simulink model "test"  (R2025b)
settings: Solver=ode5  StartTime=0.0  StopTime=40  RelTol=1e-3
StartFcn:
  | MaxMissedTicks = 99^100;
  | SampleTime = 0.01;
undefined symbols (not defined in the file or in its folder): National_Instruments, PCI
libraries: sldrtlib x6, simulink x1
settings Model: Creator=labadmin  LastModifiedBy=aie4-26
settings HardwareCC: ProdBitPerLong=64.0  ProdHWDeviceType=Intel->x86-64 (Linux 64)
settings RTWCC: SystemTargetFile=sldrt.tlc  TemplateMakefile=sldrt.tmf  RTWCompilerOptimization=on  GPUComputeCapability=3.5  Description=Simulink Desktop Real-Time
settings CodeAppCC: MaxIdLength=95.0
settings SimulinkDesktopRealTimeCC: ExtModeTransport=0.0  ExtModeStaticAllocSize=1000000.0  TargetLibSuffix=_sldrt.a  TargetPreCompLibLocation=C:\Program Files\MATLAB\R2025b\toolbox\sldrt\lib\win64  MultiwordLength=2048.0  DynamicStringBufferSize=256.0  ParMdlRefBuildCompliant=on  PreserveMATLABNamespacesInGeneratedCode=on  SubcomponentCodeInterfacePackaging=Reusable function

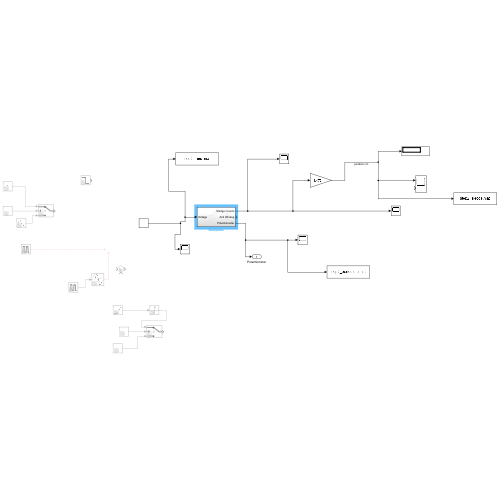
[thumbnail: Simulink's stored preview of the top-level diagram]
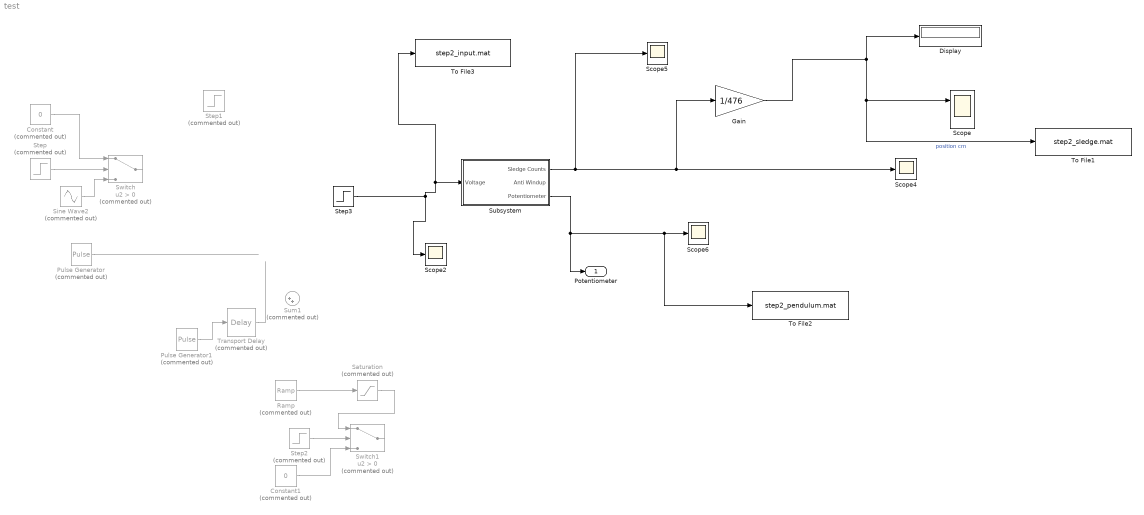
== system test ==
  Constant : Constant  Commented=on  Value=0
  Constant1 : Constant  Commented=on  Value=0
  Display : Display
  Gain : Gain  Gain=1/476
  Pulse Generator : DiscretePulseGenerator  Commented=on  PulseType=Time based  Amplitude=2  Period=10  PulseWidth=3
  Pulse Generator1 : DiscretePulseGenerator  Commented=on  PulseType=Time based  Amplitude=-2  Period=10  PulseWidth=3
  Ramp : simulink/Sources/Ramp  Commented=on  slope=-0.15  start=0  InitialOutput=0
  Saturation : Saturate  Commented=on  UpperLimit=2.2  LowerLimit=-2.2
  Scope : Scope  NumInputPorts=2
      settings: ActiveDisplayYMinimum=-17.820378151260503  ActiveDisplayYMaximum=12.400210084033613  DataLoggingVariableName=ScopeData4
  Scope{2,4..6} (4 alike) : Scope
      Scope2 settings: ActiveDisplayYMinimum=-3.223794053653696  ActiveDisplayYMaximum=6.037574387127588  DataLoggingVariableName=ScopeData6
      Scope4 settings: ActiveDisplayYMinimum=-385.49999999999989  ActiveDisplayYMaximum=3469.5  DataLoggingVariableName=ScopeData8
      Scope5 settings: ActiveDisplayYMinimum=-30594.375  ActiveDisplayYMaximum=3399.3749999999991  DataLoggingVariableName=ScopeData9
      Scope6 settings: ActiveDisplayYMinimum=1.2257068801624322  ActiveDisplayYMaximum=2.6464125172297863  DataLoggingVariableName=ScopeData10
  Sine Wave2 : Sin  Commented=on  Amplitude=1.8  Frequency=4  SampleTime=0
  Step : Step  Commented=on  Time=20  SampleTime=0
  Step1 : Step  Commented=on  Time=0.5  Before=2  After=0  SampleTime=0
  Step2 : Step  Commented=on  Time=10  Before=1  After=0  SampleTime=0
  Step3 : Step  Time=2.0  Before=1.5  After=0  SampleTime=0
  Subsystem : Subsystem
  Sum1 : Sum  Commented=on  Inputs=|++
  Switch : Switch  Commented=on  Criteria=u2 > Threshold  SaturateOnIntegerOverflow=off  InputSameDT=off
  Switch1 : Switch  Commented=on  Criteria=u2 > Threshold  SaturateOnIntegerOverflow=off  InputSameDT=off
  To File1 : ToFile  Filename=step2_sledge.mat  SaveFormat=Timeseries
  To File2 : ToFile  Filename=step2_pendulum.mat  SaveFormat=Timeseries
  To File3 : ToFile  Filename=step2_input.mat  SaveFormat=Timeseries
  Transport Delay : TransportDelay  Commented=on  DelayTime=5
  Potentiometer : Outport
  wires:
  Subsystem/1(Sledge Counts) -> Gain/1, Scope4/1, Scope5/1
  Gain/1 -> Scope/1, To File1/1, Display/1  "position cm"
  Subsystem/3(Potentiometer) -> To File2/1, Scope6/1, Potentiometer/1
  Pulse Generator1/1 -> Transport Delay/1
  Pulse Generator/1 -> ?
  Transport Delay/1 -> ?
  Step/1 -> Switch/2
  Sine Wave2/1 -> Switch/3
  Constant/1 -> Switch/1
  Step3/1 -> To File3/1, Subsystem/1(Voltage), Scope2/1
  Saturation/1 -> Switch1/1
  Step2/1 -> Switch1/2
  Ramp/1 -> Saturation/1
  Constant1/1 -> Switch1/3

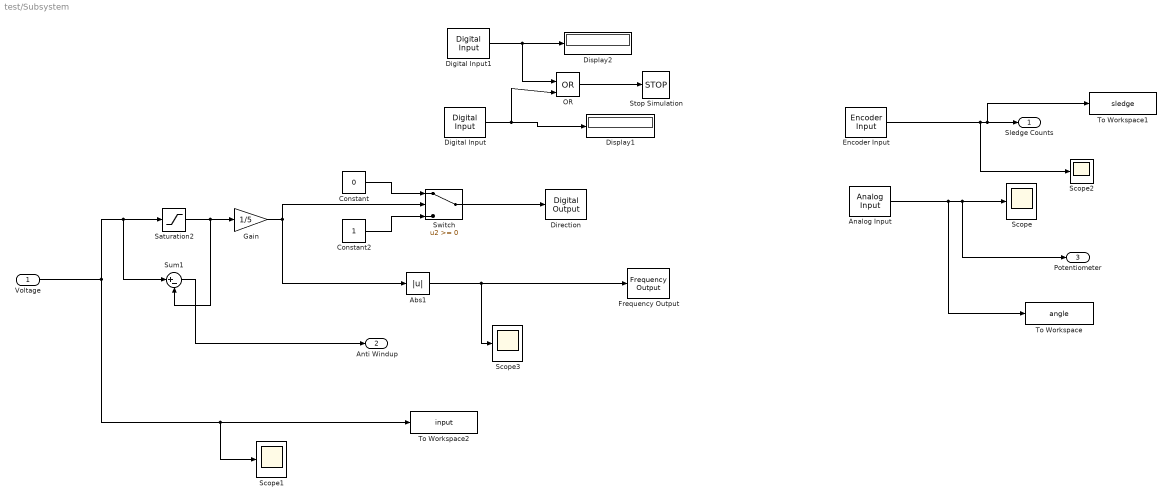
== system test/Subsystem ==
  Voltage : Inport
  Abs1 : Abs  SaturateOnIntegerOverflow=off
  Analog Input : sldrtlib/Analog Input  SampleTime=0.001  MaxMissedTicks=MaxMissedTicks  ShowMissedTicks=off  YieldWhenWaiting=off  DrvName=National_Instruments/PCI-6229  DrvAddress=4294967295  DrvOptions=[1 1 8192 2 3]  Channels=1  RangeMode=1  VoltRange=2  DataType=1
      settings: AttributesFormatString=National Instruments\nPCI-6229 [auto]
  Constant : Constant  Value=0  SampleTime=SampleTime
  Constant2 : Constant  SampleTime=SampleTime
  Digital Input : sldrtlib/Digital Input  SampleTime=0.1  MaxMissedTicks=10  ShowMissedTicks=off  YieldWhenWaiting=off  DrvName=National_Instruments/PCI-6229  DrvAddress=4294967295  DrvOptions=[1 1 8192 2 3]  Channels=2  BitMode=1  DataType=9
      settings: AttributesFormatString=National Instruments\nPCI-6229 [auto]
  Digital Input1 : sldrtlib/Digital Input  SampleTime=0.1  MaxMissedTicks=10  ShowMissedTicks=off  YieldWhenWaiting=off  DrvName=National_Instruments/PCI-6229  DrvAddress=4294967295  DrvOptions=[1 1 8192 2 3]  Channels=3  BitMode=1  DataType=9
      settings: AttributesFormatString=National Instruments\nPCI-6229 [auto]
  Direction : sldrtlib/Digital Output  SampleTime=SampleTime  MaxMissedTicks=MaxMissedTicks  ShowMissedTicks=off  YieldWhenWaiting=off  DrvName=National_Instruments/PCI-6229  DrvAddress=4294967295  DrvOptions=[1 1 8192 2 3]  Channels=1  BitMode=1  InitialValue=0  FinalValue=0
      settings: AttributesFormatString=National Instruments\nPCI-6229 [auto]
  Display1 : Display
  Display2 : Display
  Encoder Input : sldrtlib/Encoder Input  SampleTime=0.001  MaxMissedTicks=10000000  ShowMissedTicks=off  YieldWhenWaiting=off  DrvName=National_Instruments/PCI-6229  DrvAddress=4294967295  DrvOptions=[1 1 8192 2 3]  Channels=1  QuadMode=2  IndexPulse=2  InputFilter=Inf  DataType=1
      settings: AttributesFormatString=National Instruments\nPCI-6229 [auto]
  Frequency Output : sldrtlib/Frequency Output  SampleTime=SampleTime  MaxMissedTicks=MaxMissedTicks  ShowMissedTicks=off  YieldWhenWaiting=off  DrvName=National_Instruments/PCI-6229  DrvAddress=4294967295  DrvOptions=[1 1 8192 2 3]  Channels=2  FrequencySource=1  Frequency=10000  FrequencyFinalValue=[]  DutySource=2  Duty=0  DutyFinalValue=0
      settings: AttributesFormatString=National Instruments\nPCI-6229 [auto]
  Gain : Gain  Gain=1/5
  OR : Logic  Operator=OR  IconShape=distinctive  AllPortsSameDT=off  OutDataTypeStr=boolean
  Saturation2 : Saturate  UpperLimit=2.5  LowerLimit=-2.5
  Scope{,1..3} (4 alike) : Scope
      Scope settings: ActiveDisplayYMinimum=-1.7267364976437558  ActiveDisplayYMaximum=6.2920540572750241
      Scope1 settings: ActiveDisplayYMinimum=-3.75  ActiveDisplayYMaximum=3.75  DataLoggingVariableName=ScopeData2
      Scope2 settings: ActiveDisplayYMinimum=-935.75  ActiveDisplayYMaximum=8421.75  DataLoggingVariableName=ScopeData3
      Scope3 settings: ActiveDisplayYMinimum=-0.0625  ActiveDisplayYMaximum=0.5625
  Stop Simulation : Stop
  Sum1 : Sum  Inputs=|+-
  Switch : Switch  SaturateOnIntegerOverflow=off  InputSameDT=off
  To Workspace : ToWorkspace  VariableName=angle  SaveFormat=Timeseries  SampleTime=-1
  To Workspace1 : ToWorkspace  VariableName=sledge  SaveFormat=Timeseries  SampleTime=-1
  To Workspace2 : ToWorkspace  VariableName=input  SaveFormat=Timeseries  SampleTime=-1
  Sledge Counts : Outport
  Anti Windup : Outport  Port=2
  Potentiometer : Outport  Port=3
  wires:
  Digital Input/1 -> OR/2, Display1/1
  Abs1/1 -> Scope3/1, Frequency Output/1
  Constant/1 -> Switch/1
  Digital Input1/1 -> OR/1, Display2/1
  Voltage/1 -> Scope1/1, To Workspace2/1, Sum1/1, Saturation2/1
  Analog Input/1 -> To Workspace/1, Potentiometer/1, Scope/1
  OR/1 -> Stop Simulation/1
  Saturation2/1 -> Sum1/2, Gain/1
  Constant2/1 -> Switch/3
  Sum1/1 -> Anti Windup/1
  Encoder Input/1 -> Scope2/1, Sledge Counts/1, To Workspace1/1
  Switch/1 -> Direction/1
  Gain/1 -> Abs1/1, Switch/2
